simulink model "traffic_light"  (R2020a)
settings: Solver=VariableStepAuto  StartTime=0.0  StopTime=10.0  RelTol=1e-3
settings Model: Creator=Admin  LastModifiedBy=Admin

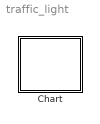
== system traffic_light ==
  Chart : Stateflow chart  TreatAsAtomicUnit=on

== stateflow chart traffic_light/Chart ==
  state stop
  state go
  state prepare_to_stop
    state yellow
  (default) -> stop
  prepare_to_stop -> stop
  stop -> go
  go -> prepare_to_stop
